simulink model "mpc_activesetqp"  (R2023a)
settings: Solver=ode45  StartTime=0.0  StopTime=40  RelTol=1e-3  EnableMultiTasking=on
values from neighbouring files (symbols this model uses):
  Ac = [1 0 0 0;       -1 0 0 0;        0 1 0 0;        0 -1 0 0;        0 0 1 0;        0 0 -1 0;        0 0 0 1;        0 0 0 -1]    [mpccustomqp1.m]
  b0 = [1;1;1;1;1;1;1;1]    [mpccustomqp1.m]
  F = CONV'*Q_hat*M    [mpccustomqp1.m]
  Linv = L\eye(size(H,1))    [mpccustomqp1.m]
  opt = mpcActiveSetOptions    [mpccustomqp1.m]
settings Model: Creator=The MathWorks, Inc.  LastModifiedBy=The MathWorks, Inc.
settings SolverCC: AlgebraicLoopSolver=TrustRegion
settings DataIOCC: LimitDataPoints=on  ReturnWorkspaceOutputs=off
settings OptimizationCC: LifeSpan=inf
settings DebuggingCC: UnconnectedInputMsg=warning  UnconnectedOutputMsg=warning  UnconnectedLineMsg=warning  AllowSymbolicDim=off  SFUnexpectedBacktrackingDiag=warning  SFNoUnconditionalDefaultTransitionDiag=warning  SFExecutionAtInitializationDiag=none  ArithmeticOperatorsInVariantConditions=warning
settings HardwareCC: ProdBitPerPointer=32  ProdBitPerSizeT=32  ProdBitPerPtrDiffT=32  ProdLargestAtomicFloat=None  ProdIntDivRoundTo=Undefined  ProdEndianess=Unspecified  ProdWordSize=32  ProdHWDeviceType=32-bit Generic
settings ModelReferenceCC: EnableRefExpFcnMdlSchedulingChecks=on  PropagateSignalLabelsOutOfModel=off
settings SFSimCC: SimUseLocalCustomCode=off  CustomCodeUndefinedFunction=UseInterfaceOnly
settings RTWCC: RTWUseLocalCustomCode=off
settings CodeAppCC: StateflowObjectComments=on
settings GRTTargetCC: TargetLangStandard=C89/C90 (ANSI)
settings ConfigComp: CovMetricSettings=dw  CovSaveCumulativeToWorkspaceVar=on  CovSaveSingleToWorkspaceVar=on  CovExternalEMLEnable=off

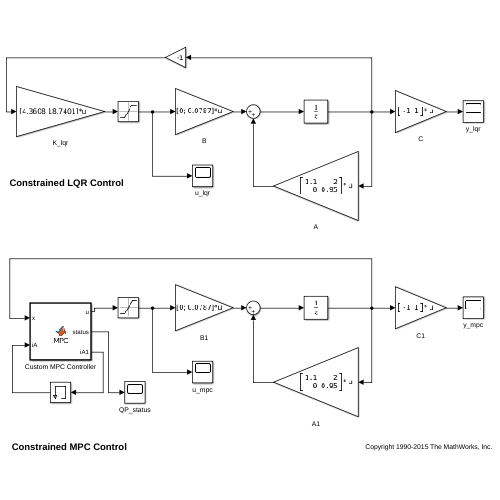
[thumbnail: Simulink's stored preview of the top-level diagram]
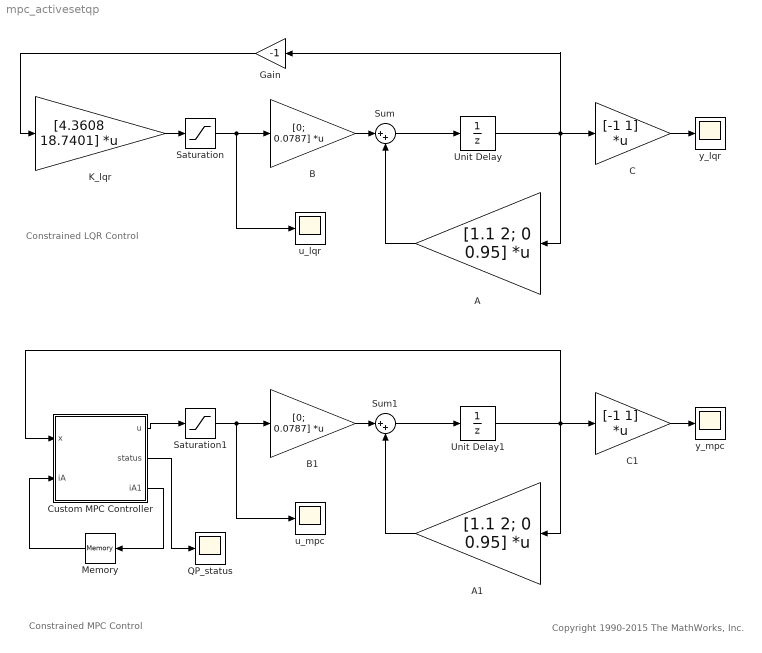
== system mpc_activesetqp ==
  note: Constrained LQR Control
  note: Constrained MPC Control
  note: Copyright 1990-2015 The MathWorks, Inc.
  A : Gain  Gain=[1.1 2; 0 0.95]  Multiplication=Matrix(K*u)
  A1 : Gain  Gain=[1.1 2; 0 0.95]  Multiplication=Matrix(K*u)
  B : Gain  Gain=[0; 0.0787]  Multiplication=Matrix(K*u)
  B1 : Gain  Gain=[0; 0.0787]  Multiplication=Matrix(K*u)
  C : Gain  Gain=[-1 1]  Multiplication=Matrix(K*u)
  C1 : Gain  Gain=[-1 1]  Multiplication=Matrix(K*u)
  Custom MPC Controller : MATLAB Function  TreatAsAtomicUnit=on
  Gain : Gain  Gain=-1
  K_lqr : Gain  Gain=[4.3608 18.7401]  Multiplication=Matrix(K*u)
  Memory : Memory  InitialCondition=false(8,1)
  QP_status : Scope
  Saturation : Saturate  UpperLimit=1  LowerLimit=-1
  Saturation1 : Saturate  UpperLimit=1  LowerLimit=-1
  Sum : Sum  Inputs=|++
  Sum1 : Sum  Inputs=|++
  Unit Delay : UnitDelay  InitialCondition=[0.5;-0.5]  HasFrameUpgradeWarning=on
  Unit Delay1 : UnitDelay  InitialCondition=[0.5;-0.5]  HasFrameUpgradeWarning=on
  u_lqr : Scope
  u_mpc : Scope
  y_lqr : Scope
  y_mpc : Scope
  wires:
  Unit Delay/1 -> Gain/1, A/1, C/1
  Sum/1 -> Unit Delay/1
  A/1 -> Sum/2
  B/1 -> Sum/1
  Saturation/1 -> u_lqr/1, B/1
  K_lqr/1 -> Saturation/1
  C/1 -> y_lqr/1
  Gain/1 -> K_lqr/1
  Sum1/1 -> Unit Delay1/1
  A1/1 -> Sum1/2
  B1/1 -> Sum1/1
  Saturation1/1 -> u_mpc/1, B1/1
  C1/1 -> y_mpc/1
  Unit Delay1/1 -> A1/1, Custom MPC Controller/1(x), C1/1
  Custom MPC Controller/1(u) -> Saturation1/1
  Custom MPC Controller/3(iA1) -> Memory/1
  Memory/1 -> Custom MPC Controller/2(iA)
  Custom MPC Controller/2(status) -> QP_status/1

== matlab function mpc_activesetqp/Custom MPC Controller ==
  settings: updateMethod=DISCRETE  sampleTime=1
  data: u output; status output; x input; iA input boolean; iA1 output; Linv parameter; F parameter; Ac parameter; b0 parameter; opt parameter
function [u,status,iA1] = MPC(x,iA,Linv,F,Ac,b0,opt)
%#codegen
[uMPC,status,iA1] = mpcActiveSetSolver(Linv,F*x,Ac,b0,[],zeros(0,1),iA,opt);
u = uMPC(1);
